simulink model "L476RG_external_mode"  (R2018b)
settings: Solver=FixedStepDiscrete  StartTime=0.0  StopTime=inf  FixedStep=0.002  RelTol=1e-3  EnableMultiTasking=on
undefined symbols (not defined in the file): L476RG, Nucleo
libraries: ADC_Lib x1, DAC_Lib x1, STM32_Config_Lib x1, TIMERS_Lib x1
settings Model: SimulationMode=external  ExtModeTrigDuration=10  Creator=The MathWorks, Inc.  LastModifiedBy=fenard1
settings DataIOCC: LimitDataPoints=on  SaveFormat=Array
settings OptimizationCC: UseDivisionForNetSlopeComputation=on  UseFloatMulNetSlope=on  UseSpecifiedMinMax=on  PassReuseOutputArgsAs=Individual arguments  ZeroExternalMemoryAtStartup=off  ZeroInternalMemoryAtStartup=off  NoFixptDivByZeroProtection=on  EfficientFloat2IntCast=on  LifeSpan=Inf  MaxStackSize=64  OptimizeBlockOrder=speed  DifferentSizesBufferReuse=on
settings DebuggingCC: SignalInfNanChecking=error  UnderspecifiedInitializationDetection=Classic  MergeDetectMultiDrivingBlocksExec=none  SolverPrmCheckMsg=warning  MultiTaskDSMMsg=none  IntegerOverflowMsg=error  AssertControl=DisableAll  AllowSymbolicDim=off  SFUnexpectedBacktrackingDiag=warning  SFNoUnconditionalDefaultTransitionDiag=warning  SFUndirectedBroadcastEventsDiag=error  SFExecutionAtInitializationDiag=none
settings HardwareCC: ProdBitPerPointer=32  ProdBitPerSizeT=32  ProdBitPerPtrDiffT=32  ProdLargestAtomicInteger=Integer  ProdWordSize=32  ProdHWDeviceType=STMicroelectronics->STM32 32-bit Cortex-M
settings ModelReferenceCC: PropagateSignalLabelsOutOfModel=off
settings SFSimCC: SimUseLocalCustomCode=off  CompileTimeRecursionLimit=0  EnableRuntimeRecursion=off  MATLABDynamicMemAlloc=off
settings RTWCC: SystemTargetFile=stm32.tlc  TLCOptions=-aInlineSetEventsForThisBaseRateFcn=TLC_FALSE  TemplateMakefile=stm32.tmf  Description=stm32 (Embedded Target)  GenerateReport=on  RTWUseLocalCustomCode=off  Toolchain=GNU Tools for ARM Embedded Processors  BuildConfiguration=Faster Runs
settings CodeAppCC: IgnoreCustomStorageClasses=off  CustomSymbolStrType=$N$R$M  StateflowObjectComments=on
settings STFCustomTargetCC: ParMdlRefBuildCompliant=on  IncludeMdlTerminateFcn=off  CombineOutputUpdateFcns=on  CombineSignalStateStructs=on  ERTCustomFileBanners=on  SupportNonFinite=off  SupportComplex=off  SupportContinuousTime=off  SupportNonInlinedSFcns=off  RemoveResetFunc=on  ParenthesesLevel=Maximum  CastingMode=Standards  MATLABClassNameForMDSCustomization=Simulink.SoftwareTarget.ERTCustomization  SystemTargetFile=stm32.tlc
settings ERTTargetCC: MultiwordLength=2048  CompOptLevelCompliant=off  ConcurrentExecutionCompliant=off  IncludeMdlTerminateFcn=off  CombineSignalStateStructs=on  SupportNonFinite=off  SupportComplex=off  ParenthesesLevel=Maximum  CastingMode=Standards  ModelStepFunctionPrototypeControlCompliant=off  CPPClassGenCompliant=off  UseToolchainInfoCompliant=off  ExtMode=on  ExtModeStaticAllocSize=256  ExtModeMexFile=ext_serial_win32_comm  ExtModeMexArgs=0,19,115200,5  ERTSrcFileBannerTemplate=sourceFileTemplate.cgt  ERTHdrFileBannerTemplate=sourceFileTemplate.cgt  ERTDataSrcFileTemplate=sourceFileTemplate.cgt  ERTDataHdrFileTemplate=sourceFileTemplate.cgt  ERTCustomFileTemplate=customRoutineProcess.tlc  EnableSignedLeftShifts=off  EnableSignedRightShifts=off
settings ConfigComp: CovMetricSettings=dw  CovHtmlReporting=on  CovSaveCumulativeToWorkspaceVar=on  CovSaveSingleToWorkspaceVar=on  CovExternalEMLEnable=off  CovSFcnEnable=off

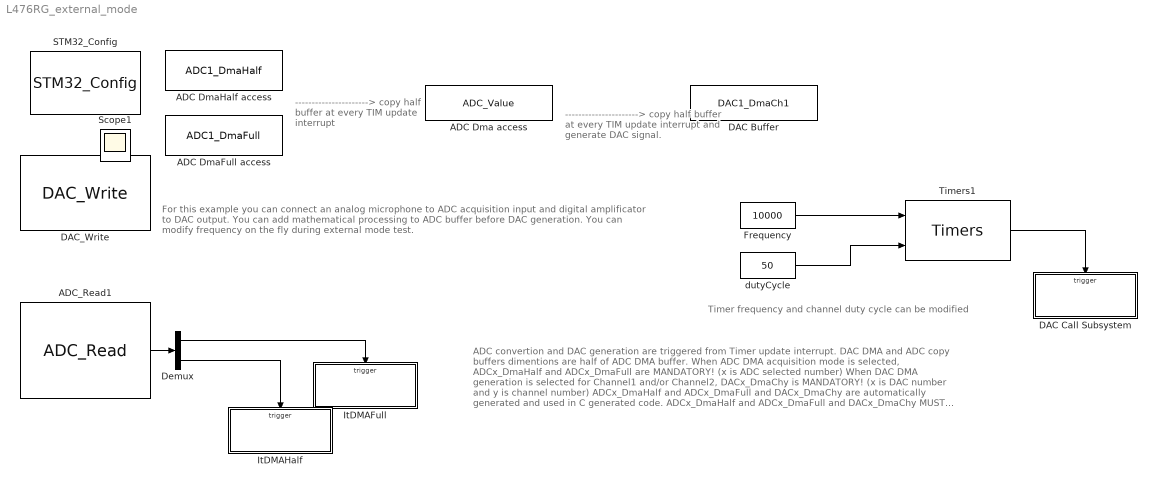
== system L476RG_external_mode ==
  note: For this example you can connect an analog microphone to ADC acquisition input
      | and digital amplificator to DAC output.
      | You can add mathematical processing to ADC buffer before DAC generation.
      | You can modify frequency on the fly during external mode test.
  note: ---------------------->
      | copy half buffer at
      | every TIM update
      | interrupt
  note: ADC convertion and DAC generation are triggered from Timer update interrupt.
      | DAC DMA and ADC copy buffers dimentions are half of ADC DMA buffer.
      |
      | When ADC DMA acquisition mode is selected, ADCx_DmaHalf and ADCx_DmaFull are MANDATORY! (x is ADC selected number)
      | When DAC DMA generation is selected for Channel1 and/or Channel2, DACx_DmaChy is MANDATORY! (x is DAC number and y is channel number)
      |
      | ADCx_DmaHalf and ADCx_DmaFull and DACx_DmaChy are automatically generated
      | and used in C generated code.
      |
      | ADCx_DmaHalf and ADCx_DmaFull and DACx_DmaChy MUST be defined as ImportedExternPointer.
  note: Timer frequency and channel duty cycle can be modified
  note: ---------------------->
      | copy half buffer at
      | every TIM update
      | interrupt and generate
      | DAC signal.
  ADC Dma access : DataStoreMemory  DataStoreName=ADC_Value  ReadBeforeWriteMsg=warning  WriteAfterWriteMsg=warning  WriteAfterReadMsg=warning  ShowAdditionalParam=off  OutDataTypeStr=uint16  Dimensions=128
  ADC DmaFull access : DataStoreMemory  DataStoreName=ADC1_DmaFull  ReadBeforeWriteMsg=warning  WriteAfterWriteMsg=warning  WriteAfterReadMsg=warning  ShowAdditionalParam=off  OutDataTypeStr=uint16  Dimensions=128
      settings: RTWStateStorageClass=ImportedExternPointer
  ADC DmaHalf access : DataStoreMemory  DataStoreName=ADC1_DmaHalf  ReadBeforeWriteMsg=warning  WriteAfterWriteMsg=warning  WriteAfterReadMsg=warning  ShowAdditionalParam=off  OutDataTypeStr=uint16  Dimensions=128
      settings: RTWStateStorageClass=ImportedExternPointer
  ADC_Read1 : ADC_Lib/ADC_Read  ADC_Name=ADC1  ADC_Ch0=off  ADC_Ch1=off  ADC_Ch2=off  ADC_Ch3=off  ADC_Ch4=off  ADC_Ch5=off  ADC_Ch6=off  ADC_Ch7=off  ADC_Ch8=off  ADC_Ch9=off  ADC_Ch10=off  ADC_Ch11=off  ADC_Ch12=off  ADC_Ch13=off  ADC_Ch14=off  ADC_Ch15=off  ADC_Ch16=off  ADC_Ch17=off  ADC_Ch18=off  RgRk1=off  RgRk2=off  RgRk3=off  RgRk4=off  RgRk1_Ch=Ch15_r1  RgRk2_Ch=off  RgRk3_Ch=off  RgRk4_Ch=off  RgRk5=off  RgRk6=off  RgRk7=off  RgRk8=off  RgRk5_Ch=off  RgRk6_Ch=off  RgRk7_Ch=off  RgRk8_Ch=off  RgRk9=off  RgRk10=off  RgRk11=off  RgRk12=off  RgRk9_Ch=off  RgRk10_Ch=off  RgRk11_Ch=off  RgRk12_Ch=off  RgRk13=off  RgRk14=off  RgRk15=off  RgRk16=off  RgRk13_Ch=off  RgRk14_Ch=off  RgRk15_Ch=off  RgRk16_Ch=off  InjRk1=off  InjRk2=off  InjRk3=off  InjRk4=off  InjRk1_Ch=off  InjRk2_Ch=off  InjRk3_Ch=off  InjRk4_Ch=off  ADC_Trig=T2_TRGO  ADC_TrigEdge=RISING  DmaReq=on  DMA_Buffer=256  ItReq=on  AWD_Mode=NOT_USED  AWD_Ch=0  AWD_HThres=0  AWD_LThres=0  AWD_En_Int=off  AWD2_HThres=0  AWD2_LThres=0  AWD2_En_Int=off  AWD3_HThres=0  AWD3_LThres=0  AWD3_En_Int=off  EOC_SEQ=on  EOC_IT=off  JEOC_IT=off  AWD_IT=off  OVR_IT=off  CpltTrans=on  HalfTrans=on  ADC_RegNb=1  ADC_RegCh0=off  ADC_RegCh1=off  ADC_RegCh2=off  ADC_RegCh3=off  ADC_RegCh4=off  ADC_RegCh5=off  ADC_RegCh6=off  ADC_RegCh7=off  ADC_RegCh8=off  ADC_RegCh9=off  ADC_RegCh10=off  ADC_RegCh11=off  ADC_RegCh12=off  ADC_RegCh13=off  ADC_RegCh14=off  ADC_RegCh15=on  ADC_RegCh16=off  ADC_RegCh17=off  ADC_RegCh18=off  ADC_InjNb=0  ADC_InjCh0=off  ADC_InjCh1=off  ADC_InjCh2=off  ADC_InjCh3=off  ADC_InjCh4=off  ADC_InjCh5=off  ADC_InjCh6=off  ADC_InjCh7=off  ADC_InjCh8=off  ADC_InjCh9=off  ADC_InjCh10=off  ADC_InjCh11=off  ADC_InjCh12=off  ADC_InjCh13=off  ADC_InjCh14=off  ADC_InjCh15=off  ADC_InjCh16=off  ADC_InjCh17=off  ADC_InjCh18=off  NbADC=1  CurrentADC=ADC1
      settings: SourceProductName=Target Support Package - STM32 Adapter
  DAC Buffer : DataStoreMemory  DataStoreName=DAC1_DmaCh1  ReadBeforeWriteMsg=warning  WriteAfterWriteMsg=warning  WriteAfterReadMsg=warning  ShowAdditionalParam=off  OutDataTypeStr=uint16  Dimensions=128
      settings: RTWStateStorageClass=ImportedExternPointer
  DAC Call Subsystem : Subsystem  TreatAsAtomicUnit=on
  DAC_Write : DAC_Lib/DAC_Write  DAC_Name=DAC1  Pin0=off  Pin1=off  Align=12bit_right  DmaBuffCh1=128  DmaBuffCh2=0  CpltTrans=off  HalfTrans=off  ErrorIt=off  UnderIt=off  NbDAC=1  UsedDma=on
      settings: SourceProductName=Target Support Package - STM32 Adapter
  Demux : Demux  Outputs=2
  Frequency : Constant  Value=10000
  ItDMAFull : Subsystem  TreatAsAtomicUnit=on
  ItDMAHalf : Subsystem  TreatAsAtomicUnit=on
  STM32_Config : STM32_Config_Lib/STM32_Config  Priority=0  Project_Path=.\  Config_File=L476RG-Nucleo.ioc  MCU_Name=STM32L476RGTx
      settings: SourceProductName=Target Support Package - STM32 Adapter
  Timers1 : TIMERS_Lib/Timers  currentTIM=TIM2  TIM_Name=TIM2  sysUsingTimer=on  TIM_APBClock=80000000  TIM_Set_Clk=off  TIM_Prescaler=3  TIM_Clock=20000000.00  Variable_frequency=on  TIM_Set_OutFreq=on  TIM_ARR=2000  Output_frequency=10000.00  Repetition_counter=0  TIM_Mode=Up  TIM_DMA=none  TIM_IRQ=on  TIM_IRQ_ONLY=off  TIM_UP=on  TIM_TRG=off  TIM_COM=off  TIM_BRK=off  NbTIM=1  CH1_enable=on  CH1N_enable=off  CH1_type=Output_PWM  CH1_DMA=off  CH1_int=off  CH1_edge=Rising  CH1_div=1  CH1_variable_duty=on  CH1_set_pulse=on  CH1_output_duty=50  CH1_pulse=1000  CH2_enable=off  CH2N_enable=off  CH2_type=Output_PWM  CH2_DMA=off  CH2_int=off  CH2_edge=Rising  CH2_div=1  CH2_variable_duty=off  CH2_set_pulse=off  CH2_output_duty=0.00  CH2_pulse=0  CH3_enable=off  CH3N_enable=off  CH3_type=Unknown  CH3_DMA=off  CH3_int=off  CH3_edge=Rising  CH3_div=1  CH3_variable_duty=off  CH3_set_pulse=off  CH3_output_duty=0.00  CH3_pulse=0  CH4_enable=off  CH4N_enable=off  CH4_type=Unknown  CH4_DMA=off  CH4_int=off  CH4_edge=Rising  CH4_div=1  CH4_variable_duty=off  CH4_set_pulse=off  CH4_output_duty=0.00  CH4_pulse=0
      settings: SourceProductName=Target Support Package - STM32 Adapter
  dutyCycle : Constant  Value=50
  Scope1 : Scope
  wires:
  Timers1/1 -> DAC Call Subsystem/Trigger
  ADC_Read1/1 -> Demux/1
  Demux/1 -> ItDMAFull/Trigger
  Demux/2 -> ItDMAHalf/Trigger
  Frequency/1 -> Timers1/1
  dutyCycle/1 -> Timers1/2

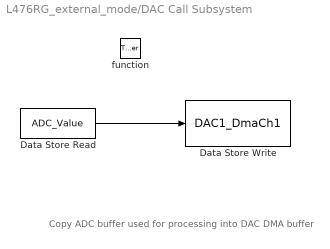
== system L476RG_external_mode/DAC Call Subsystem ==
  note: Copy ADC buffer used for processing into DAC DMA buffer
  function : TriggerPort  TriggerType=function-call  VariantControl=Variant
  Data Store Read : DataStoreRead  DataStoreName=ADC_Value
  Data Store Write : DataStoreWrite  DataStoreName=DAC1_DmaCh1
  wires:
  Data Store Read/1 -> Data Store Write/1

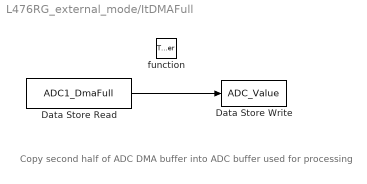
== system L476RG_external_mode/ItDMAFull ==
  note: Copy second half of ADC DMA buffer into ADC buffer used for processing
  function : TriggerPort  TriggerType=function-call  VariantControl=Variant
  Data Store Read : DataStoreRead  DataStoreName=ADC1_DmaFull
  Data Store Write : DataStoreWrite  DataStoreName=ADC_Value
  wires:
  Data Store Read/1 -> Data Store Write/1

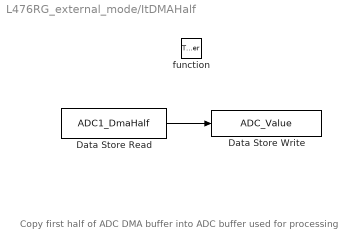
== system L476RG_external_mode/ItDMAHalf ==
  note: Copy first half of ADC DMA buffer into ADC buffer used for processing
  function : TriggerPort  TriggerType=function-call  VariantControl=Variant
  Data Store Read : DataStoreRead  DataStoreName=ADC1_DmaHalf
  Data Store Write : DataStoreWrite  DataStoreName=ADC_Value
  wires:
  Data Store Read/1 -> Data Store Write/1
